simulink model "AFU_20b"  (R2022a)
settings: Solver=FixedStepAuto  StartTime=0.0  StopTime=Inf  FixedStep=1/100  RelTol=1e-3
PostLoadFcn:
  | Pos_Cmd = 0;
  | Vel_Cmd = 0;
  | Psi_Cmd = 0;
  | Psid_Cmd = 0;
  | Throttle = 0;
  | Steer = 0;
  | LatLon_deg = [36;42];
  | LatLon = LatLon_deg*pi/180;
libraries: etargetslib x2, shared6dof x1, simulink x1, simulink_extras x1, slrealtimeiplib x1
settings Model: Creator=afuzunkaya  LastModifiedBy=Pc
settings SolverCC: AlgebraicLoopSolver=TrustRegion
settings DataIOCC: SaveOutput=off  SignalLogging=off  DSMLogging=off  SaveTime=off  ReturnWorkspaceOutputs=off
settings ModelReferenceCC: EnableRefExpFcnMdlSchedulingChecks=off
settings RTWCC: Description=Generic Real-Time Target  DLArmComputeVersion=19.05

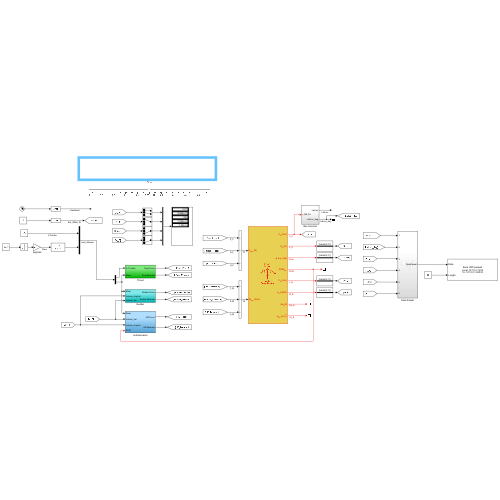
[thumbnail: Simulink's stored preview of the top-level diagram]
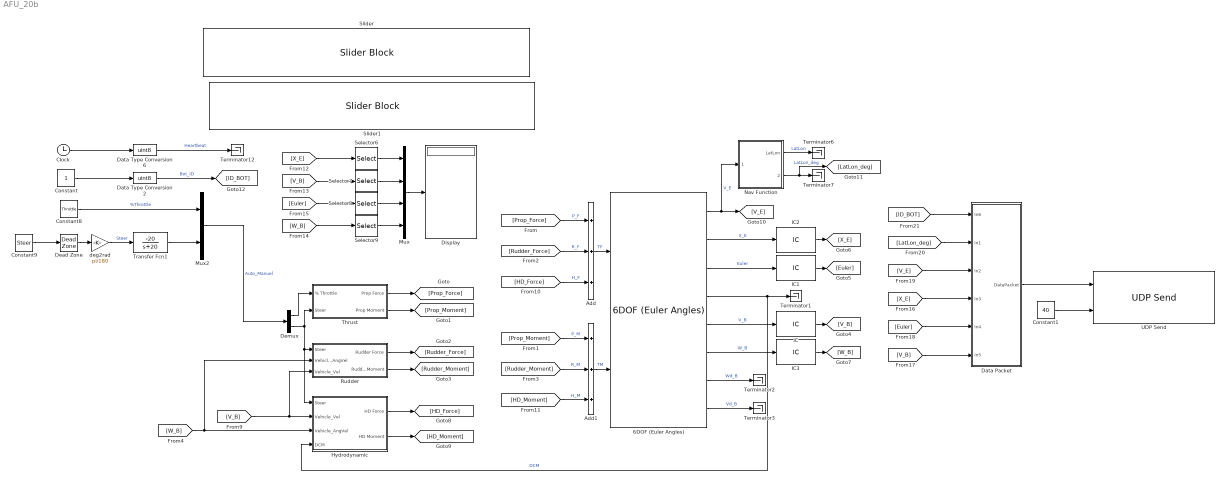
== system AFU_20b ==
  6DOF (Euler Angles) : shared6dof/6DOF (Euler Angles)  units=Metric (MKS)  mtype=Fixed  rep=Euler Angles  xme_0=[0 0 0]  Vm_0=[0 0 0]  eul_0=[0 0 0]  pm_0=[0 0 0]  mass_0=250  mass_e=0.5  mass_f=2.0  inertia=eye(3)*15  inertia_e=eye(3)  inertia_f=2*eye(3)  k_quat=1.0  vre_flag=on  abi_flag=off  aMode=0  xme_statename=''  Vm_statename=''  eul_statename=''  quat_statename=''  pm_statename=''  mass_statename=''
      settings: SourceProductBaseCode=AE,PW,DR,MT,VE
  Add : Sum  Inputs=+++
  Add1 : Sum  Inputs=+++
  Clock : Clock
  Constant : Constant
  Constant1 : Constant  Value=40
  Constant8 : Constant  Value=Throttle
  Constant9 : Constant  Value=Steer
  Data Packet : Subsystem
  Data Type Conversion2 : DataTypeConversion  OutDataTypeStr=uint8  RndMeth=Nearest  SaturateOnIntegerOverflow=off
  Data Type Conversion6 : DataTypeConversion  OutDataTypeStr=uint8  RndMeth=Nearest
  Dead Zone : DeadZone  LowerValue=-0.01  UpperValue=0.01
  Demux : Demux  Outputs=2
  Display : Display
  Hydrodynamic : Subsystem
  IC{,1..3} (4 alike) : InitialCondition  Value=zeros(3,1)
  Mux : Mux
  Mux2 : Mux  Inputs=2
  Nav Function : Subsystem
  Rudder : Subsystem
  Selector6 : Selector  InputPortWidth=3  IndexOptions=Index vector (dialog)  Indices=[1 2]  OutputSizes=1
  Selector7 : Selector  InputPortWidth=3  IndexOptions=Index vector (dialog)  Indices=1  OutputSizes=1
  Selector8 : Selector  InputPortWidth=3  IndexOptions=Index vector (dialog)  Indices=3  OutputSizes=1
  Selector9 : Selector  InputPortWidth=3  IndexOptions=Index vector (dialog)  Indices=3  OutputSizes=1
  Slider : SliderBlock  ScaleMin=-100  TickInterval=25
  Slider1 : SliderBlock  ScaleMin=-1  ScaleMax=1  TickInterval=0.2
  Terminator{1..3,6..7,12} (6 alike) : Terminator
  Thrust : Subsystem
  Transfer Fcn1 : TransferFcn  Numerator=-20  Denominator=[1 20]
  UDP Send : slrealtimeiplib/UDP Send  useHostTargetConn=off  toAddress=127.0.0.1  toPort=22333  sampleTime=0.01*2  enableMessage=off  ipAddress=127.0.0.1  localPort=222
      settings: SourceProductBaseCode=XP
  deg2rad : Gain  Gain=pi/180
  wires:
  Thrust/1(Prop Force) -> [Prop_Force]
  Thrust/2(Prop Moment) -> [Prop_Moment]
  [Prop_Force] -> Add/1  "P_F"
  [Prop_Moment] -> Add1/1  "P_M"
  Add1/1 -> 6DOF (Euler Angles)/2  "TM"
  [Rudder_Moment] -> Add1/2  "R_M"
  Rudder/2(Rudder Moment) -> [Rudder_Moment]
  Rudder/1(Rudder Force) -> [Rudder_Force]
  [Rudder_Force] -> Add/2  "R_F"
  6DOF (Euler Angles)/5 -> IC/1  "V_B"
  IC/1 -> [V_B]
  IC1/1 -> [Euler]
  6DOF (Euler Angles)/3 -> IC1/1  "Euler"
  IC2/1 -> [X_E]
  6DOF (Euler Angles)/2 -> IC2/1  "X_E"
  6DOF (Euler Angles)/6 -> IC3/1  "W_B"
  6DOF (Euler Angles)/1 -> [V_E], Nav Function/1(v_BE_Fe)  "V_E"
  6DOF (Euler Angles)/4 -> Hydrodynamic/4(DCM), Terminator1/1  "DCM"
  6DOF (Euler Angles)/7 -> Terminator2/1  "Wd_B"
  6DOF (Euler Angles)/8 -> Terminator3/1  "Vd_B"
  [V_B] -> Rudder/3(Vehicle_Vel), Hydrodynamic/2(Vehicle_Vel)
  Hydrodynamic/1(HD Force) -> [HD_Force]
  Hydrodynamic/2(HD Moment) -> [HD_Moment]
  [HD_Force] -> Add/3  "H_F"
  [HD_Moment] -> Add1/3  "H_M"
  [X_E] -> Selector6/1
  [V_B] -> Selector7/1
  Selector9/1 -> Mux/4
  Selector8/1 -> Mux/3
  [Euler] -> Selector8/1
  [W_B] -> Selector9/1
  Selector6/1 -> Mux/1
  Selector7/1 -> Mux/2
  Mux/1 -> Display/1
  Demux/1 -> Thrust/1(% Throttle)
  Demux/2 -> Hydrodynamic/1(Steer), Rudder/1(Steer), Thrust/2(Steer)
  Constant8/1 -> Mux2/1  "%Throttle"
  Constant9/1 -> Dead Zone/1
  Transfer Fcn1/1 -> Mux2/2
  deg2rad/1 -> Transfer Fcn1/1  "Steer"
  [W_B] -> Rudder/2(Vehicle_AngVel), Hydrodynamic/3(Vehicle_AngVel)
  Nav Function/2(LatLon_deg) -> [LatLon_deg], Terminator7/1  "LatLon_deg"
  Nav Function/1(LatLon) -> Terminator6/1  "LatLon"
  Dead Zone/1 -> deg2rad/1
  Constant1/1 -> UDP Send/2
  Add/1 -> 6DOF (Euler Angles)/1  "TF"
  IC3/1 -> [W_B]
  Data Type Conversion2/1 -> [ID_BOT]  "Bot_ID"
  Constant/1 -> Data Type Conversion2/1
  Clock/1 -> Data Type Conversion6/1
  Data Type Conversion6/1 -> Terminator12/1  "Heartbeat"
  [LatLon_deg] -> Data Packet/2(In1)
  [V_E] -> Data Packet/3(In2)
  [X_E] -> Data Packet/4(In3)
  [Euler] -> Data Packet/5(In4)
  [V_B] -> Data Packet/6(In5)
  Data Packet/1(DataPacket) -> UDP Send/1
  [ID_BOT] -> Data Packet/1(In6)
  Mux2/1 -> Demux/1  "Auto_Manuel"

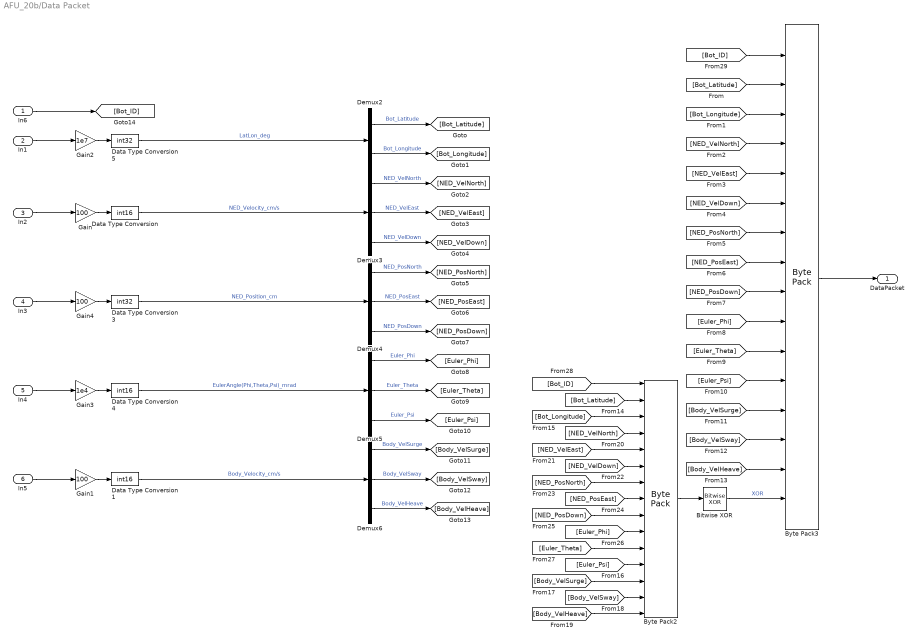
== system AFU_20b/Data Packet ==
  In6 : Inport
  In1 : Inport  Port=2
  In2 : Inport  Port=3
  In3 : Inport  Port=4
  In4 : Inport  Port=5
  In5 : Inport  Port=6
  Bitwise XOR : simulink/Logic and Bit Operations/Bitwise Operator  logicop=XOR  UseBitMask=off  BitMask=bin2dec('11011001')  BitMaskRealWorld=Stored Integer
  Byte Pack2 : etargetslib/Byte Pack  datatypes={'uint8','int32','int32','int16','int16','int16','int32','int32','int32','int16','int16','int16','int16','int16','int16'}  byteAlign=1
  Byte Pack3 : etargetslib/Byte Pack  datatypes={'uint8','int32','int32','int16','int16','int16','int32','int32','int32','int16','int16','int16','int16','int16','int16','uint8'}  byteAlign=1
  Data Type Conversion : DataTypeConversion  OutDataTypeStr=int16  RndMeth=Nearest  SaturateOnIntegerOverflow=off
  Data Type Conversion1 : DataTypeConversion  OutDataTypeStr=int16  RndMeth=Nearest  SaturateOnIntegerOverflow=off
  Data Type Conversion3 : DataTypeConversion  OutDataTypeStr=int32  RndMeth=Nearest  SaturateOnIntegerOverflow=off
  Data Type Conversion4 : DataTypeConversion  OutDataTypeStr=int16  RndMeth=Nearest  SaturateOnIntegerOverflow=off
  Data Type Conversion5 : DataTypeConversion  OutDataTypeStr=int32  RndMeth=Nearest  SaturateOnIntegerOverflow=off
  Demux2 : Demux  Outputs=2
  Demux{3..6} (4 alike) : Demux  Outputs=3
  Gain : Gain  Gain=100
  Gain1 : Gain  Gain=100
  Gain2 : Gain  Gain=1e7
  Gain3 : Gain  Gain=1e4
  Gain4 : Gain  Gain=100
  DataPacket : Outport
  wires:
  Data Type Conversion/1 -> Demux3/1  "NED_Velocity_cm/s"
  In5/1 -> Gain1/1
  Data Type Conversion1/1 -> Demux6/1  "Body_Velocity_cm/s"
  Gain2/1 -> Data Type Conversion5/1
  Gain1/1 -> Data Type Conversion1/1
  Data Type Conversion3/1 -> Demux4/1  "NED_Position_cm"
  Demux2/1 -> [Bot_Latitude]  "Bot_Latitude"
  Gain3/1 -> Data Type Conversion4/1
  Demux3/1 -> [NED_VelNorth]  "NED_VelNorth"
  Gain4/1 -> Data Type Conversion3/1
  Gain/1 -> Data Type Conversion/1
  In1/1 -> Gain2/1
  Demux2/2 -> [Bot_Longitude]  "Bot_Longitude"
  In4/1 -> Gain3/1
  Data Type Conversion4/1 -> Demux5/1  "EulerAngle(Phi,Theta,Psi)_mrad"
  Data Type Conversion5/1 -> Demux2/1  "LatLon_deg"
  In2/1 -> Gain/1
  In3/1 -> Gain4/1
  Byte Pack2/1 -> Bitwise XOR/1
  Byte Pack3/1 -> DataPacket/1
  Bitwise XOR/1 -> Byte Pack3/16  "XOR"
  Demux3/2 -> [NED_VelEast]  "NED_VelEast"
  Demux3/3 -> [NED_VelDown]  "NED_VelDown"
  Demux4/1 -> [NED_PosNorth]  "NED_PosNorth"
  Demux4/2 -> [NED_PosEast]  "NED_PosEast"
  Demux4/3 -> [NED_PosDown]  "NED_PosDown"
  Demux5/1 -> [Euler_Phi]  "Euler_Phi"
  Demux5/2 -> [Euler_Theta]  "Euler_Theta"
  Demux5/3 -> [Euler_Psi]  "Euler_Psi"
  Demux6/1 -> [Body_VelSurge]  "Body_VelSurge"
  Demux6/2 -> [Body_VelSway]  "Body_VelSway"
  Demux6/3 -> [Body_VelHeave]  "Body_VelHeave"
  [Bot_Latitude] -> Byte Pack3/2
  [Bot_Longitude] -> Byte Pack3/3
  [NED_VelNorth] -> Byte Pack3/4
  [NED_VelEast] -> Byte Pack3/5
  [NED_VelDown] -> Byte Pack3/6
  [NED_PosNorth] -> Byte Pack3/7
  [NED_PosEast] -> Byte Pack3/8
  [NED_PosDown] -> Byte Pack3/9
  [Euler_Phi] -> Byte Pack3/10
  [Euler_Theta] -> Byte Pack3/11
  [Euler_Psi] -> Byte Pack3/12
  [Body_VelSurge] -> Byte Pack3/13
  [Body_VelSway] -> Byte Pack3/14
  [Body_VelHeave] -> Byte Pack3/15
  [Bot_Latitude] -> Byte Pack2/2
  [Bot_Longitude] -> Byte Pack2/3
  [NED_VelNorth] -> Byte Pack2/4
  [NED_VelEast] -> Byte Pack2/5
  [NED_VelDown] -> Byte Pack2/6
  [NED_PosNorth] -> Byte Pack2/7
  [NED_PosEast] -> Byte Pack2/8
  [Euler_Phi] -> Byte Pack2/10
  [Body_VelSway] -> Byte Pack2/14
  [Body_VelHeave] -> Byte Pack2/15
  [Body_VelSurge] -> Byte Pack2/13
  [Euler_Psi] -> Byte Pack2/12
  [Euler_Theta] -> Byte Pack2/11
  [NED_PosDown] -> Byte Pack2/9
  In6/1 -> [Bot_ID]
  [Bot_ID] -> Byte Pack2/1
  [Bot_ID] -> Byte Pack3/1

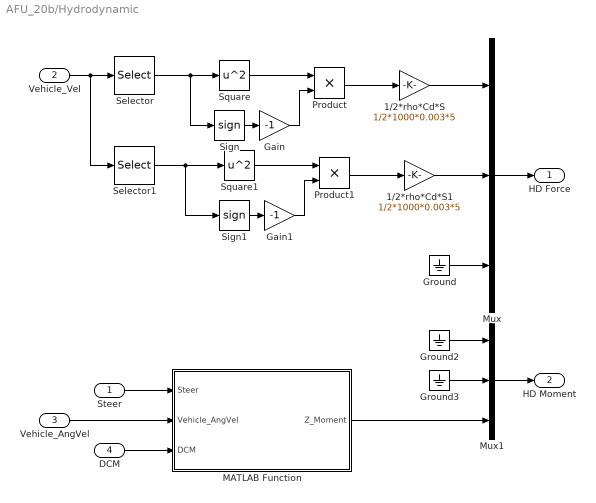
== system AFU_20b/Hydrodynamic ==
  Steer : Inport
  Vehicle_Vel : Inport  Port=2
  Vehicle_AngVel : Inport  Port=3
  DCM : Inport  Port=4
  1/2*rho*Cd*S : Gain  Gain=1/2*1000*0.003*5
  1/2*rho*Cd*S1 : Gain  Gain=1/2*1000*0.003*5
  Gain : Gain  Gain=-1
  Gain1 : Gain  Gain=-1
  Ground : Ground
  Ground2 : Ground
  Ground3 : Ground
  MATLAB Function : MATLAB Function  TreatAsAtomicUnit=on
  Mux : Mux  Inputs=3
  Mux1 : Mux  Inputs=3
  Product : Product
  Product1 : Product
  Selector : Selector  InputPortWidth=3  IndexOptions=Index vector (dialog)  Indices=1  OutputSizes=1
  Selector1 : Selector  InputPortWidth=3  IndexOptions=Index vector (dialog)  Indices=2  OutputSizes=1
  Sign : Signum
  Sign1 : Signum
  Square : Math  Operator=square
  Square1 : Math  Operator=square
  HD Force : Outport
  HD Moment : Outport  Port=2
  wires:
  Vehicle_Vel/1 -> Selector1/1, Selector/1
  Square/1 -> Product/1
  1/2*rho*Cd*S1/1 -> Mux/2
  Mux/1 -> HD Force/1
  Ground3/1 -> Mux1/2
  Ground2/1 -> Mux1/1
  Mux1/1 -> HD Moment/1
  1/2*rho*Cd*S/1 -> Mux/1
  Sign/1 -> Gain/1
  Product/1 -> 1/2*rho*Cd*S/1
  Gain/1 -> Product/2
  Selector/1 -> Square/1, Sign/1
  Selector1/1 -> Sign1/1, Square1/1
  Gain1/1 -> Product1/2
  Product1/1 -> 1/2*rho*Cd*S1/1
  Sign1/1 -> Gain1/1
  Square1/1 -> Product1/1
  Vehicle_AngVel/1 -> MATLAB Function/2(Vehicle_AngVel)
  Ground/1 -> Mux/3
  Steer/1 -> MATLAB Function/1(Steer)
  MATLAB Function/1(Z_Moment) -> Mux1/3
  DCM/1 -> MATLAB Function/3(DCM)

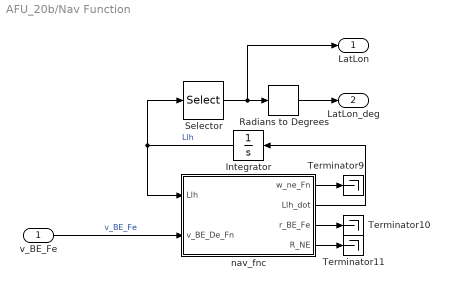
== system AFU_20b/Nav Function ==
  v_BE_Fe : Inport
  Integrator : Integrator  InitialCondition=[LatLon;0]  WrapState=on  WrappedStateUpperValue=[pi;pi;Inf]  WrappedStateLowerValue=[-pi;-pi;-Inf]
  Radians to Degrees : simulink_extras/Transformations/Radians to Degrees
  Selector : Selector  InputPortWidth=3  IndexOptions=Index vector (dialog)  Indices=[1 2]  OutputSizes=1
  Terminator10 : Terminator
  Terminator11 : Terminator
  Terminator9 : Terminator
  nav_fnc : MATLAB Function  TreatAsAtomicUnit=on
  LatLon : Outport  VectorParamsAs1DForOutWhenUnconnected=off
  LatLon_deg : Outport  Port=2  VectorParamsAs1DForOutWhenUnconnected=off
  wires:
  nav_fnc/1(w_ne_Fn) -> Terminator9/1
  nav_fnc/3(r_BE_Fe) -> Terminator10/1
  nav_fnc/4(R_NE) -> Terminator11/1
  nav_fnc/2(Llh_dot) -> Integrator/1
  Integrator/1 -> nav_fnc/1(Llh), Selector/1  "Llh"
  v_BE_Fe/1 -> nav_fnc/2(v_BE_De_Fn)  "v_BE_Fe"
  Selector/1 -> LatLon/1, Radians to Degrees/1
  Radians to Degrees/1 -> LatLon_deg/1

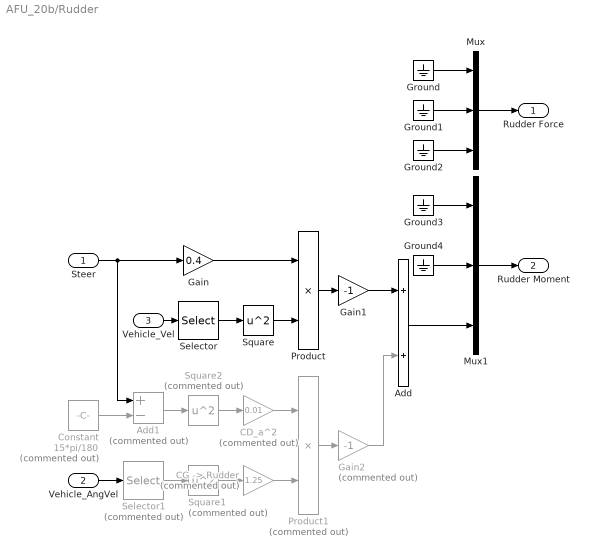
== system AFU_20b/Rudder ==
  Steer : Inport
  Vehicle_AngVel : Inport  Port=2
  Vehicle_Vel : Inport  Port=3
  Add : Sum
  Add1 : Sum  Commented=on  Inputs=+-
  CD_a^2 : Gain  Commented=on  Gain=0.01
  "CG -> Rudder" : Gain  Commented=on  Gain=1.25
  Constant : Constant  Commented=on  Value=15*pi/180
  Gain : Gain  Gain=0.4
  Gain1 : Gain  Gain=-1
  Gain2 : Gain  Commented=on  Gain=-1
  Ground{,1..4} (5 alike) : Ground
  Mux : Mux  Inputs=3
  Mux1 : Mux  Inputs=3
  Product : Product
  Product1 : Product  Commented=on
  Selector : Selector  InputPortWidth=3  IndexOptions=Index vector (dialog)  Indices=1  OutputSizes=1
  Selector1 : Selector  Commented=on  InputPortWidth=3  IndexOptions=Index vector (dialog)  Indices=3  OutputSizes=1
  Square : Math  Operator=square
  Square1 : Math  Commented=on  Operator=square
  Square2 : Math  Commented=on  Operator=square
  Rudder Force : Outport
  Rudder Moment : Outport  Port=2
  wires:
  Mux1/1 -> Rudder Moment/1
  Ground3/1 -> Mux1/1
  Ground4/1 -> Mux1/2
  Product/1 -> Gain1/1
  Mux/1 -> Rudder Force/1
  Ground2/1 -> Mux/3
  Ground1/1 -> Mux/2
  Ground/1 -> Mux/1
  Vehicle_Vel/1 -> Selector/1
  Square/1 -> Product/2
  Gain/1 -> Product/1
  Selector/1 -> Square/1
  Add/1 -> Mux1/3
  Vehicle_AngVel/1 -> Selector1/1
  "CG -> Rudder"/1 -> Product1/2
  Square1/1 -> "CG -> Rudder"/1
  Constant/1 -> Add1/2
  Add1/1 -> Square2/1
  Square2/1 -> CD_a^2/1
  CD_a^2/1 -> Product1/1
  Product1/1 -> Gain2/1
  Gain2/1 -> Add/2
  Selector1/1 -> Square1/1
  Gain1/1 -> Add/1
  Steer/1 -> Add1/1, Gain/1

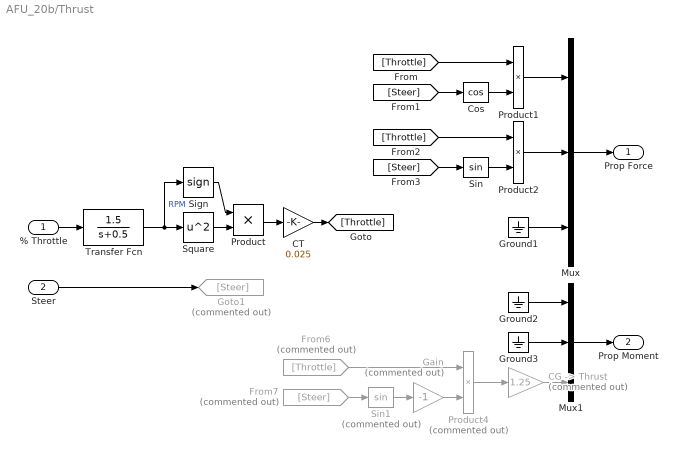
== system AFU_20b/Thrust ==
  % Throttle : Inport
  Steer : Inport  Port=2
  "CG -> Thrust" : Gain  Commented=on  Gain=1.25
  CT : Gain  Gain=0.025
  Cos : Trigonometry  Operator=cos
  From6 : From  Commented=on  GotoTag=Throttle
  From7 : From  Commented=on  GotoTag=Steer
  Gain : Gain  Commented=on  Gain=-1
  Goto1 : Goto  Commented=on  GotoTag=Steer
  Ground1 : Ground
  Ground2 : Ground
  Ground3 : Ground
  Mux : Mux  Inputs=3
  Mux1 : Mux  Inputs=3
  Product : Product
  Product1 : Product
  Product2 : Product
  Product4 : Product  Commented=on
  Sign : Signum
  Sin : Trigonometry
  Sin1 : Trigonometry  Commented=on
  Square : Math  Operator=square
  Transfer Fcn : TransferFcn  Numerator=[1.5]  Denominator=[1 0.5]
  Prop Force : Outport
  Prop Moment : Outport  Port=2
  wires:
  % Throttle/1 -> Transfer Fcn/1
  Transfer Fcn/1 -> Sign/1, Square/1  "RPM"
  Square/1 -> Product/2
  CT/1 -> [Throttle]
  Product2/1 -> Mux/2
  Ground1/1 -> Mux/3
  Mux/1 -> Prop Force/1
  "CG -> Thrust"/1 -> Mux1/3
  Ground3/1 -> Mux1/2
  Ground2/1 -> Mux1/1
  Mux1/1 -> Prop Moment/1
  Sign/1 -> Product/1
  Product/1 -> CT/1
  [Steer] -> Cos/1
  Cos/1 -> Product1/2
  Product1/1 -> Mux/1
  [Throttle] -> Product1/1
  [Throttle] -> Product2/1
  Sin/1 -> Product2/2
  [Steer] -> Sin/1
  From7/1 -> Sin1/1
  Sin1/1 -> Gain/1
  From6/1 -> Product4/1
  Product4/1 -> "CG -> Thrust"/1
  Gain/1 -> Product4/2
  Steer/1 -> Goto1/1

== matlab function AFU_20b/Hydrodynamic/MATLAB Function ==
  data: Steer input; Z_Moment output; Vehicle_AngVel input; DCM input
function Z_Moment = fcn(Steer, Vehicle_AngVel, DCM)

if abs(Steer) <= 0.01
   w_be_Fe = DCM.'*Vehicle_AngVel;
   Z_Moment = -5*w_be_Fe(3);
else
   Z_Moment = Vehicle_AngVel(3)^2*-1*sign(Vehicle_AngVel(3))* (1/2*1000*0.003*5);
end

== matlab function AFU_20b/Nav Function/nav_fnc ==
  data: Llh input; w_ne_Fn output; v_BE_De_Fn input; Llh_dot output; r_BE_Fe output; R_NE output
function [w_ne_Fn,Llh_dot,r_BE_Fe,R_NE] = nav_fnc(Llh,v_BE_De_Fn)
%#codegen

vN = v_BE_De_Fn(1);
vE = v_BE_De_Fn(2);
vD = v_BE_De_Fn(3);

L = Llh(1);
l = Llh(2);
h = Llh(3);

cL = cos(L);
sL = sin(L);
cl = cos(l);
sl = sin(l);
tL = sL/cL;

[~,~,R_N,R_E,~,~,~,e] = earthParam_rad(L);
R_NE = [R_N;R_E];

% Titterton2004 (Eq 3.87) corrected (OR Groves2008 5.37, Farrell2008 11.41)
w_ne_Fn_1 = vE/(R_E + h);
w_ne_Fn = [
     w_ne_Fn_1;
    -vN/(R_N + h);
    -w_ne_Fn_1*tL;
];

% Titterton2004 (Eq.s 3.85, 3.86, 3.81)
Llh_dot = [
    -w_ne_Fn(2);
     w_ne_Fn_1/cL;
    -vD;
];

% Groves2008 2.70
r_BE_Fe = [
    (R_E + h)*cL*cl;
    (R_E + h)*cL*sl;
    ((1 - e^2)*R_E + h)*sL;
];

function [w_earth,R0,R_N,R_E,R,r,f,e,t_srd] = earthParam_rad(L)
%earthParam  Return navigational parameters of the earth
%==========================================================================
%   [w_earth,R0,R_N,R_E,R,r,f,e] = earthParam(L,unit)
%       This is the low-level function called by "earthParam" that supports
%       code generation. "exist" and "convang" functions are extracted to 
%       this function's caller "earthParam".
%
%       Function's I/O definition is a subset of that of earthParam's.
%       Type "help earthParam" for further explanation on function's usage.

%   Author       : spakkan
%   Release date : 21.09.2018

w_earth = 7.292115e-5;

if nargout == 1
    return
end

% Titterton2004 p.52
R = 6378137;
r = 6356752.3142;
f = (R - r)/R;
e = sqrt(f*(2-f));

% Titterton2004 (Eq.s 3.83, 3.84)
den = sqrt(1 - e^2*sin(L).^2);
R_N = R*(1 - e^2)./den.^3;
R_E = R./den;
R0 = sqrt(R_N.*R_E);

t_srd = 23*3600 + 56*60 + 4.1;
